simulink model "RTS_15km"  (R2018a)
settings: Solver=ode15s  StartTime=0.0  StopTime=10  FixedStep=0.00001  RelTol=1e-3  AbsTol=1e-6
undefined symbols (not defined in the file): C1, Cline, g, K0, K2, Kline, M, Mline
libraries: simulink x3, simulink_extras x2
settings Model: Creator=FoR  LastModifiedBy=gct14001
settings SolverCC: SolverResetMethod=Robust
settings CodeAppCC: StateflowObjectComments=on

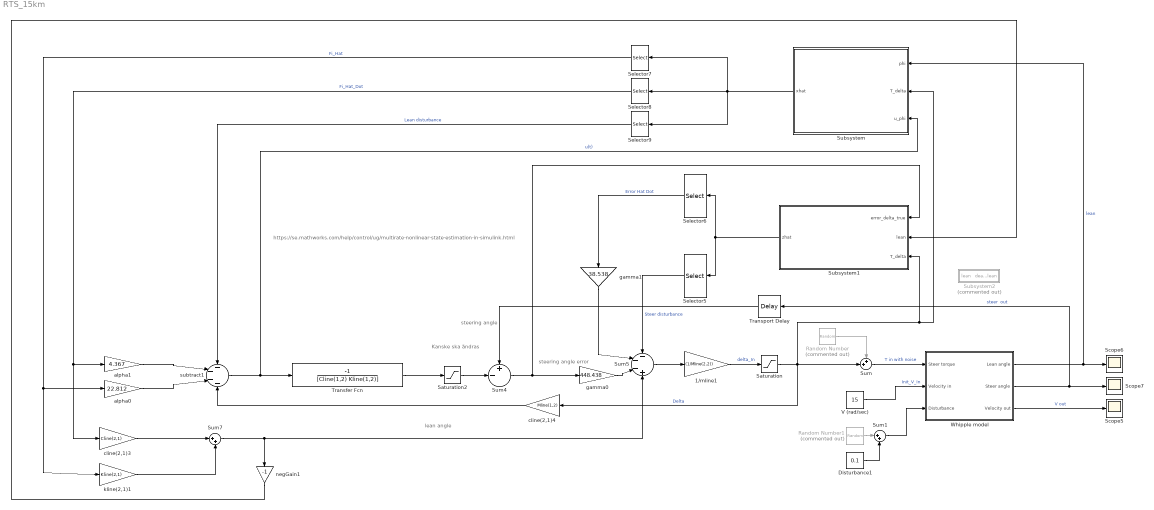
== system RTS_15km ==
  note: steering angle
  note: https://se.mathworks.com/help/control/ug/multirate-nonlinear-state-estimation-in-simulink.html
  note: steering angle error
  note: Kanske ska
      | ändras
  note: lean angle
  1/mline1 : Gain  Gain=(1/Mline(2,2))
  Disturbance1 : Constant  Value=0.1
  Random Number : RandomNumber  Commented=on  Variance=0.1  SampleTime=0.1
  Random Number1 : RandomNumber  Commented=on  Variance=0.1  SampleTime=0.1
  Saturation : Saturate  UpperLimit=12  LowerLimit=-12
  Saturation2 : Saturate  UpperLimit=90  LowerLimit=-90
  Scope5 : Scope
  Scope6 : Scope
  Scope7 : Scope
  Selector5 : Selector  InputPortWidth=6  IndexOptions=Index vector (dialog)  Indices=3  OutputSizes=1
  Selector6 : Selector  InputPortWidth=6  IndexOptions=Index vector (dialog)  Indices=2  OutputSizes=1
  Selector7 : Selector  InputPortWidth=3  IndexOptions=Index vector (dialog)  Indices=1  OutputSizes=1
  Selector8 : Selector  InputPortWidth=3  IndexOptions=Index vector (dialog)  Indices=2  OutputSizes=1
  Selector9 : Selector  InputPortWidth=3  IndexOptions=Index vector (dialog)  Indices=3  OutputSizes=1
  Subsystem : Subsystem
  Subsystem1 : Subsystem
  Subsystem2 : Subsystem  Commented=on
  Sum : Sum  Inputs=++|
  Sum1 : Sum  Inputs=|++
  Sum4 : Sum  Inputs=+-|
  Sum5 : Sum  Inputs=---+
  Sum7 : Sum  Inputs=|++
  Transfer Fcn : TransferFcn  Numerator=[-1]  Denominator=[Cline(1,2) Kline(1,2)]
  Transport Delay : TransportDelay  DelayTime=0.005
  V (rad/sec) : Constant  Value=15
  Whipple model : Subsystem
  alpha0 : Gain  Gain=22.812
  alpha1 : Gain  Gain=4.367
  cline(2,1)3 : Gain  Gain=Cline(2,1)
  cline(2,1)4 : Gain  Gain=Mline(1,2)
  gamma0 : Gain  Gain=448.438
  "gamma1 " : Gain  Gain=38.538
  kline(2,1)1 : Gain  Gain=Kline(2,1)
  negGain1 : Gain  Gain=-1
  subtract1 : Sum  Inputs=----
  wires:
  Saturation/1 -> Sum/2, cline(2,1)4/1, Subsystem1/3(T_delta), Subsystem/2(T_delta)  "Delta"
  Subsystem1/1(zhat) -> Selector5/1, Selector6/1
  Selector7/1 -> kline(2,1)1/1, alpha0/1  "Fi_Hat"
  cline(2,1)3/1 -> Sum7/1
  Selector9/1 -> subtract1/1  "Lean disturbance"
  cline(2,1)4/1 -> subtract1/4
  Selector5/1 -> Sum5/1  "Steer disturbance"
  Sum7/1 -> negGain1/1, Sum5/4
  Sum5/1 -> 1/mline1/1
  alpha0/1 -> subtract1/3
  alpha1/1 -> subtract1/2
  gamma0/1 -> Sum5/3
  kline(2,1)1/1 -> Sum7/2
  subtract1/1 -> Transfer Fcn/1, Subsystem/3(u_phi)  "u(t)"
  1/mline1/1 -> Saturation/1  "delta_In"
  Selector8/1 -> cline(2,1)3/1, alpha1/1  "Fi_Hat_Dot"
  Whipple model/3(Velocity out) -> Scope5/1  "V out"
  "gamma1 "/1 -> Sum5/2
  Sum4/1 -> Subsystem1/1(error_delta_true), gamma0/1
  Selector6/1 -> "gamma1 "/1  "Error Hat Dot"
  Saturation2/1 -> Sum4/2
  negGain1/1 -> Subsystem1/2(lean)
  Subsystem/1(xhat) -> Selector9/1, Selector8/1, Selector7/1
  V (rad/sec)/1 -> Whipple model/2(Velocity in)  "Init_V_In"
  Whipple model/2(Steer angle) -> Scope7/1, Transport Delay/1  "steer  out"
  Transfer Fcn/1 -> Saturation2/1
  Transport Delay/1 -> Sum4/1
  Sum/1 -> Whipple model/1(Steer torque)  "T in with noise"
  Random Number/1 -> Sum/1
  Whipple model/1("Lean angle ") -> Subsystem/1(phi), Scope6/1  "lean"
  Sum1/1 -> Whipple model/3(Disturbance)
  Random Number1/1 -> Sum1/1
  Disturbance1/1 -> Sum1/2

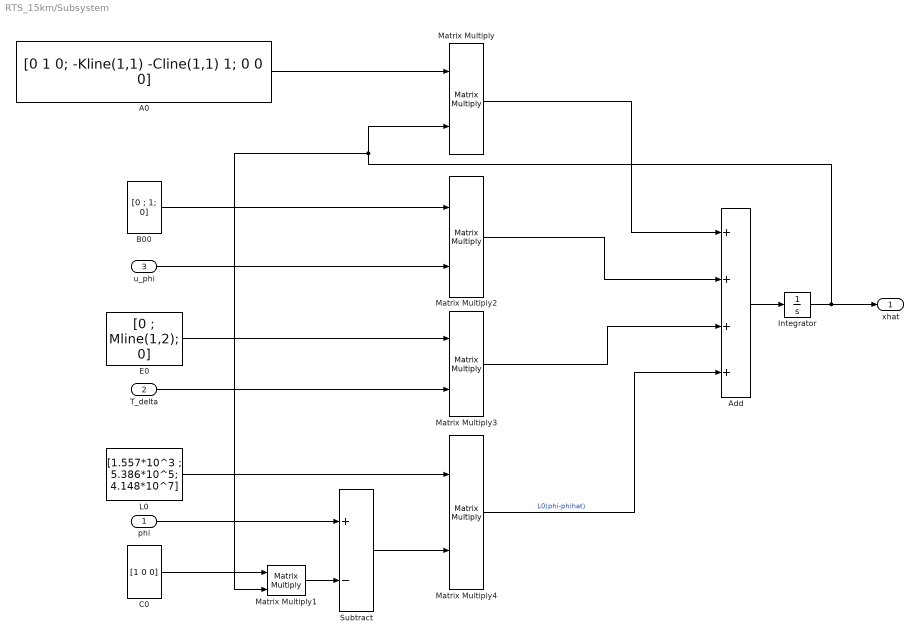
== system RTS_15km/Subsystem ==
  phi : Inport
  T_delta : Inport  Port=2
  u_phi : Inport  Port=3
  A0 : Constant  Value=[0 1 0; -Kline(1,1) -Cline(1,1) 1; 0 0 0]
  Add : Sum  Inputs=++++
  B00 : Constant  Value=[0 ; 1; 0]  VectorParams1D=off
  C0 : Constant  Value=[1 0 0]  VectorParams1D=off
  "E0 " : Constant  Value=[0 ; Mline(1,2); 0]  VectorParams1D=off
  Integrator : Integrator
  L0 : Constant  Value=[1.557*10^3 ; 5.386*10^5; 4.148*10^7]  VectorParams1D=off
  Matrix Multiply{,1..4} (5 alike) : Product  Multiplication=Matrix(*)
  Subtract : Sum  Inputs=+-
  xhat : Outport
  wires:
  A0/1 -> Matrix Multiply/1
  B00/1 -> Matrix Multiply2/1
  u_phi/1 -> Matrix Multiply2/2
  "E0 "/1 -> Matrix Multiply3/1
  T_delta/1 -> Matrix Multiply3/2
  C0/1 -> Matrix Multiply1/1
  Matrix Multiply1/1 -> Subtract/2
  phi/1 -> Subtract/1
  Subtract/1 -> Matrix Multiply4/2
  L0/1 -> Matrix Multiply4/1
  Matrix Multiply/1 -> Add/1
  Matrix Multiply2/1 -> Add/2
  Matrix Multiply3/1 -> Add/3
  Matrix Multiply4/1 -> Add/4  "L0(phi-phihat)"
  Add/1 -> Integrator/1
  Integrator/1 -> xhat/1, Matrix Multiply1/2, Matrix Multiply/2

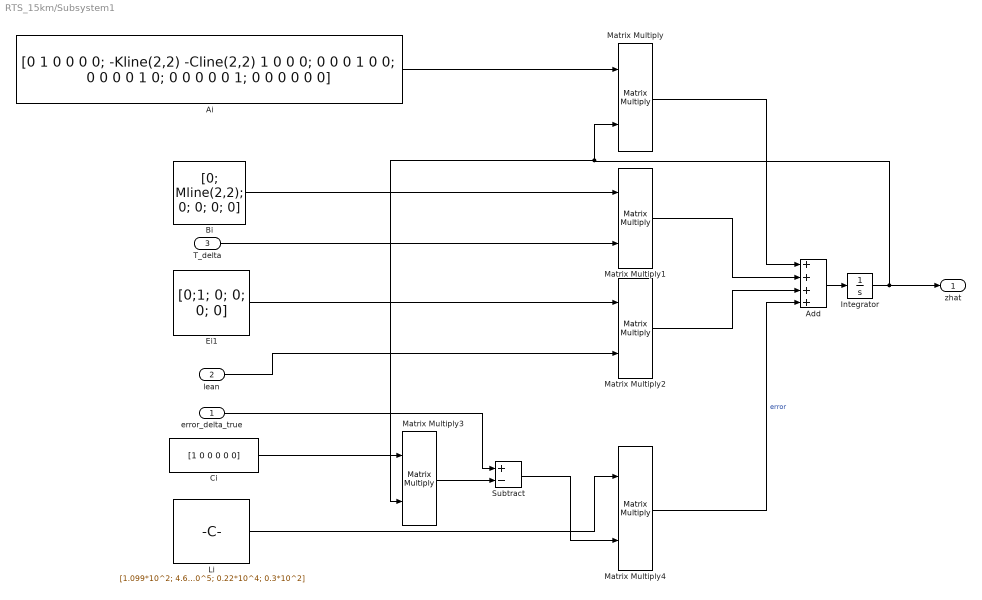
== system RTS_15km/Subsystem1 ==
  error_delta_true : Inport
  lean : Inport  Port=2
  T_delta : Inport  Port=3
  Add : Sum  Inputs=++++
  Ai : Constant  Value=[0 1 0 0 0 0; -Kline(2,2) -Cline(2,2) 1 0 0 0; 0 0 0 1 0 0; 0 0 0 0 1 0; 0 0 0 0 0 1; 0 0 0 0 0 0]
  Bi : Constant  Value=[0; Mline(2,2); 0; 0; 0; 0]  VectorParams1D=off
  Ci : Constant  Value=[1 0 0 0 0 0]  VectorParams1D=off
  Ei1 : Constant  Value=[0;1; 0; 0; 0; 0]  VectorParams1D=off
  Integrator : Integrator
  Li : Constant  Value=[1.099*10^2; 4.693*10^3; 1.094*10^5; 0.22*10^5; 0.22*10^4; 0.3*10^2]  VectorParams1D=off
  Matrix Multiply{,1..4} (5 alike) : Product  Multiplication=Matrix(*)
  Subtract : Sum  Inputs=+-
  zhat : Outport
  wires:
  T_delta/1 -> Matrix Multiply1/2
  Bi/1 -> Matrix Multiply1/1
  Ai/1 -> Matrix Multiply/1
  Ei1/1 -> Matrix Multiply2/1
  lean/1 -> Matrix Multiply2/2
  Matrix Multiply/1 -> Add/1
  Matrix Multiply1/1 -> Add/2
  Matrix Multiply2/1 -> Add/3
  Ci/1 -> Matrix Multiply3/1
  error_delta_true/1 -> Subtract/1
  Matrix Multiply3/1 -> Subtract/2
  Matrix Multiply4/1 -> Add/4  "error"
  Subtract/1 -> Matrix Multiply4/2
  Li/1 -> Matrix Multiply4/1
  Add/1 -> Integrator/1
  Integrator/1 -> Matrix Multiply3/2, Matrix Multiply/2, zhat/1

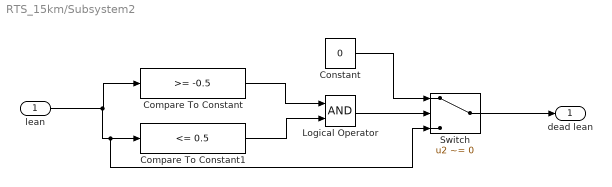
== system RTS_15km/Subsystem2 ==
  lean : Inport
  Compare To Constant : simulink/Logic and Bit Operations/Compare To Constant  relop=>=  const=-0.5  OutDataTypeStr=boolean
  Compare To Constant1 : simulink/Logic and Bit Operations/Compare To Constant  relop=<=  const=0.5  OutDataTypeStr=boolean
  Constant : Constant  Value=0
  Logical Operator : Logic  AllPortsSameDT=off  OutDataTypeStr=boolean
  Switch : Switch  Criteria=u2 ~= 0
  dead lean : Outport
  wires:
  Switch/1 -> dead lean/1
  Compare To Constant1/1 -> Logical Operator/2
  lean/1 -> Switch/3, Compare To Constant1/1, Compare To Constant/1
  Logical Operator/1 -> Switch/2
  Compare To Constant/1 -> Logical Operator/1
  Constant/1 -> Switch/1

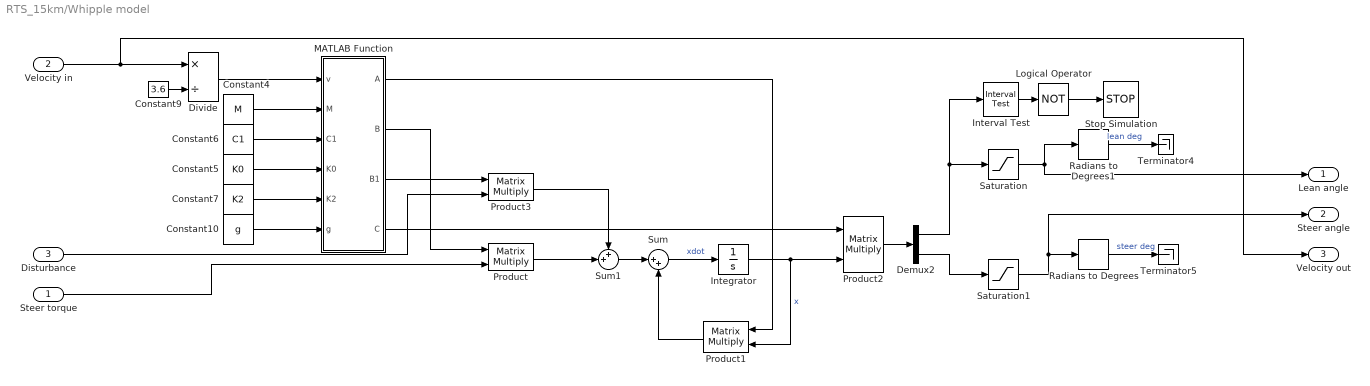
== system RTS_15km/Whipple model ==
  Steer torque : Inport
  Velocity in : Inport  Port=2
  Disturbance : Inport  Port=3
  Constant10 : Constant  Value=g
  Constant4 : Constant  Value=M
  Constant5 : Constant  Value=K0
  Constant6 : Constant  Value=C1
  Constant7 : Constant  Value=K2
  Constant9 : Constant  Value=3.6
  Demux2 : Demux  Outputs=2
  Divide : Product  Inputs=*/
  Integrator : Integrator
  Interval Test : simulink/Logic and Bit Operations/Interval Test  IntervalClosedRight=on  uplimit=pi/4  IntervalClosedLeft=on  lowlimit=-pi/4  OutDataTypeStr=boolean
  Logical Operator : Logic  Operator=NOT  AllPortsSameDT=off  OutDataTypeStr=boolean
  MATLAB Function : MATLAB Function  TreatAsAtomicUnit=on
  Product{,1..3} (4 alike) : Product  Multiplication=Matrix(*)
  Radians to Degrees : simulink_extras/Transformations/Radians to Degrees
  Radians to Degrees1 : simulink_extras/Transformations/Radians to Degrees
  Saturation : Saturate  UpperLimit=pi/2  LowerLimit=-pi/2
  Saturation1 : Saturate  UpperLimit=pi/2  LowerLimit=-pi/2
  Stop Simulation : Stop
  Sum : Sum  Inputs=|++
  Sum1 : Sum  Inputs=++|
  Terminator4 : Terminator
  Terminator5 : Terminator
  "Lean angle " : Outport
  Steer angle : Outport  Port=2
  Velocity out : Outport  Port=3
  wires:
  Saturation/1 -> "Lean angle "/1, Radians to Degrees1/1
  Saturation1/1 -> Steer angle/1, Radians to Degrees/1
  Velocity in/1 -> Velocity out/1, Divide/1
  Demux2/1 -> Interval Test/1, Saturation/1
  Product/1 -> Sum1/2
  Product1/1 -> Sum/2
  Constant7/1 -> MATLAB Function/5(K2)
  MATLAB Function/2(B) -> Product/1
  Demux2/2 -> Saturation1/1
  Constant4/1 -> MATLAB Function/2(M)
  Radians to Degrees1/1 -> Terminator4/1  "lean deg"
  Sum/1 -> Integrator/1  "xdot"
  Constant5/1 -> MATLAB Function/4(K0)
  Sum1/1 -> Sum/1
  Constant6/1 -> MATLAB Function/3(C1)
  Disturbance/1 -> Product3/2
  Interval Test/1 -> Logical Operator/1
  Product2/1 -> Demux2/1
  Constant9/1 -> Divide/2
  Integrator/1 -> Product1/2, Product2/2  "x"
  Product3/1 -> Sum1/1
  MATLAB Function/3(B1) -> Product3/1
  Logical Operator/1 -> Stop Simulation/1
  MATLAB Function/1(A) -> Product1/1
  MATLAB Function/4(C) -> Product2/1
  Divide/1 -> MATLAB Function/1(v)
  Steer torque/1 -> Product/2
  Radians to Degrees/1 -> Terminator5/1  "steer deg"
  Constant10/1 -> MATLAB Function/6(g)

== matlab function RTS_15km/Whipple model/MATLAB Function ==
  data: v input; A output; B output; B1 output; C output; M input; C1 input; K0 input; K2 input; g input
function [A,B,B1,C] = fcn(v, M, C1, K0, K2, g)

 %A matrix
 A1=[0 0; 0 0];
 A2=[1 0; 0 1];
 A3=-inv(M)*(g*K0+v^2*K2);
 A4=-inv(M)*v*C1;
 A=[A1, A2; A3, A4];
 
 %B matrix
 B=[[0; 0]; inv(M)*[0;1]]; 
 
 %B1 matrix
 B1=[[0; 0]; inv(M)*[1;0]]; 
  
 %C matrix
 C=[1 0 0 0; 0 1 0 0];
 
 %D matrix
 D=[0; 0];
